simulink model "three_way_newest_1"  (R2025b)
settings: Solver=VariableStepAuto  StartTime=0.0  StopTime=20  RelTol=1e-3
undefined symbols (not defined in the file or in its folder): c, dspblkCoreblockFVToolHelper, gcbh, sfvc784, xck26
libraries: hdlBasic x131, hdlDSPIP x11, simulink x10, hdlUtilities x4, vmcUtilities x1
(part 2 of 2)

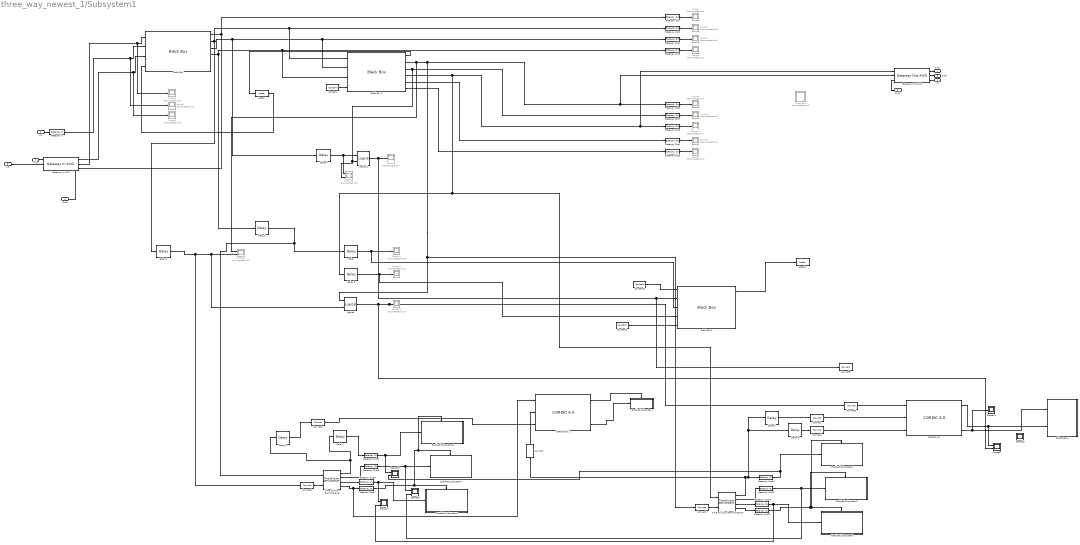
== system three_way_newest_1/Subsystem1 ==
  In1 : Inport
  In2 : Inport  Port=2
  In3 : Inport  Port=3
  In4 : Inport  Port=4
  Assert : hdlBasic/Assert  assert_type=on  type_source=Explicitly  gui_display_data_type=Fixed-point  arith_type=Unsigned  n_bits=1  bin_pt=0  preci_type=Single  exp_width=8  frac_width=24  assert_rate=on  rate_source=Explicitly  period=1/81000  output_port=on  XmcBlockStatus=1  maskContainerNames=group1  block_type=assert  block_config=sysgen:assert_config  block_width=609  block_height=900
  Assert1 : hdlBasic/Assert  assert_type=on  type_source=Explicitly  gui_display_data_type=Fixed-point  arith_type=Unsigned  n_bits=1  bin_pt=0  preci_type=Single  exp_width=8  frac_width=24  assert_rate=on  rate_source=Explicitly  period=1/81000  output_port=on  XmcBlockStatus=1  maskContainerNames=group1  block_type=assert  block_config=sysgen:assert_config  block_width=609  block_height=900
  Black Box : hdlBasic/Black Box  init_code=fir_compiler_0_wrapper_config  sim_method=Vivado Simulator  verbose=off  XmcBlockStatus=1  maskContainerNames=group1  block_type=blackbox2  block_config=sysgen:black_box_config
  Black Box1 : hdlBasic/Black Box  init_code=fir_compiler_1_wrapper_config  sim_method=Vivado Simulator  verbose=off  XmcBlockStatus=1  maskContainerNames=group1  block_type=blackbox2  block_config=sysgen:black_box_config
  Black Box2 : hdlBasic/Black Box  init_code=cordic_0_wrapper_config  sim_method=Vivado Simulator  verbose=off  XmcBlockStatus=1  maskContainerNames=group1  block_type=blackbox2  block_config=sysgen:black_box_config
  "CORDIC 6.0 " : hdlDSPIP/CORDIC 6.0   functional_selection=Translate  architectural_configuration=Parallel  pipelining_mode=Maximum  data_format=SignedFraction  phase_format=Radians  input_width=16  output_width=16  round_mode=Nearest_Even  iterations=0  precision=0  compensation_scaling=BRAM  coarse_rotation=on  aclken=off  aresetn=off  out_tready=off  cartesian_has_tuser=off  cartesian_has_tlast=off  cartesian_tuser_width=1  phase_has_tuser=off  phase_has_tlast=off  phase_tuser_width=1  out_tlast_behv=Null  flow_control=NonBlocking  optimize_goal=Resources  trim_axipin_name=on  simulation_type=hybrid_sim  simulation_model=sysgen:cordic_v6_0  data_path_portlist={'s_axis_cartesian_tdata_imag', 's_axis_cartesian_tdata_real', 's_axis_phase_tdata_phase', 'm_axis_dout_tdata_imag', 'm_axis_dout_tdata_real', 'm_axis_dout_tdata_phase','m_axis_dout_tdata'}  ip_name=CORDIC  ip_version=6.0  dsptool_ready=true  ipcore_usecache=true  ipcore_useipmodelcache=true  wrapper_available=true  port_translation_map={ 'aclken' => 'en', 'aresetn' => 'rst' }  XmcBlockStatus=1  maskContainerNames=group15  block_type=cordic_v6_0  block_config=sysgen:rodinimport_config  block_width=800
  CORDIC 6.0 1 : hdlDSPIP/CORDIC 6.0   functional_selection=Translate  architectural_configuration=Parallel  pipelining_mode=Maximum  data_format=SignedFraction  phase_format=Radians  input_width=16  output_width=16  round_mode=Nearest_Even  iterations=0  precision=0  compensation_scaling=BRAM  coarse_rotation=on  aclken=off  aresetn=off  out_tready=off  cartesian_has_tuser=off  cartesian_has_tlast=off  cartesian_tuser_width=1  phase_has_tuser=off  phase_has_tlast=off  phase_tuser_width=1  out_tlast_behv=Null  flow_control=NonBlocking  optimize_goal=Resources  trim_axipin_name=on  simulation_type=hybrid_sim  simulation_model=sysgen:cordic_v6_0  data_path_portlist={'s_axis_cartesian_tdata_imag', 's_axis_cartesian_tdata_real', 's_axis_phase_tdata_phase', 'm_axis_dout_tdata_imag', 'm_axis_dout_tdata_real', 'm_axis_dout_tdata_phase','m_axis_dout_tdata'}  ip_name=CORDIC  ip_version=6.0  dsptool_ready=true  ipcore_usecache=true  ipcore_useipmodelcache=true  wrapper_available=true  port_translation_map={ 'aclken' => 'en', 'aresetn' => 'rst' }  XmcBlockStatus=1  maskContainerNames=group15  block_type=cordic_v6_0  block_config=sysgen:rodinimport_config  block_width=800
  Constant : hdlBasic/Constant  const=1.0  gui_display_data_type=Boolean  arith_type=Boolean  n_bits=16  bin_pt=14  preci_type=Single  exp_width=8  frac_width=24  explicit_period=off  period=1  XmcBlockStatus=1  maskContainerNames=tabcontainer1  block_type=constant  block_config=sysgen:Constant_config
  Constant1 : hdlBasic/Constant  const=1.0  gui_display_data_type=Boolean  arith_type=Boolean  n_bits=16  bin_pt=14  preci_type=Single  exp_width=8  frac_width=24  explicit_period=off  period=1  XmcBlockStatus=1  maskContainerNames=tabcontainer1  block_type=constant  block_config=sysgen:Constant_config
  Constant2 : hdlBasic/Constant  const=1.0  gui_display_data_type=Boolean  arith_type=Boolean  n_bits=16  bin_pt=14  preci_type=Single  exp_width=8  frac_width=24  explicit_period=off  period=1  XmcBlockStatus=1  maskContainerNames=tabcontainer1  block_type=constant  block_config=sysgen:Constant_config
  Convert{,2,4,7} (4 alike) : hdlBasic/Convert  gui_display_data_type=Fixed-point  arith_type=Signed (2's comp)  n_bits=16  bin_pt=14  float_type=Single  exp_bits=8  fraction_bits=24  quantization="Round  (unbiased: +/- Inf)"  overflow=Saturate  en=off  latency=0  pipeline=off  XmcBlockStatus=1  maskContainerNames=group2  block_type=convert  block_config=sysgen:Convert_config  block_width=595  block_height=885
  Convert{1,3,5..6} (4 alike) : hdlBasic/Convert  gui_display_data_type=Boolean  arith_type=Boolean  n_bits=16  bin_pt=14  float_type=Single  exp_bits=8  fraction_bits=24  quantization=Truncate  overflow=Wrap  en=off  latency=0  pipeline=off  XmcBlockStatus=1  maskContainerNames=group2  block_type=convert  block_config=sysgen:Convert_config  block_width=595  block_height=885
  Delay{,3,5..6} (4 alike) : hdlBasic/Delay  rst=off  en=off  latency=1  reg_retiming=off  XmcBlockStatus=1  maskContainerNames=group1  block_type=delay  block_config=sysgen:Delay_config
  Delay1 : hdlBasic/Delay  rst=off  en=off  latency=30  reg_retiming=off  XmcBlockStatus=1  maskContainerNames=group1  block_type=delay  block_config=sysgen:Delay_config
  Delay2 : hdlBasic/Delay  rst=off  en=off  latency=30  reg_retiming=off  XmcBlockStatus=1  maskContainerNames=group1  block_type=delay  block_config=sysgen:Delay_config
  Delay4 : hdlBasic/Delay  rst=off  en=off  latency=30  reg_retiming=off  XmcBlockStatus=1  maskContainerNames=group1  block_type=delay  block_config=sysgen:Delay_config
  Delay7 : hdlBasic/Delay  rst=off  en=off  latency=267  reg_retiming=off  XmcBlockStatus=1  maskContainerNames=group1  block_type=delay  block_config=sysgen:Delay_config
  Delay8 : hdlBasic/Delay  rst=off  en=off  latency=267  reg_retiming=off  XmcBlockStatus=1  maskContainerNames=group1  block_type=delay  block_config=sysgen:Delay_config
  Enabled Subsystem : Subsystem  TreatAsAtomicUnit=on
  Enabled Subsystem1 : Subsystem  TreatAsAtomicUnit=on
  Enabled Subsystem2 : Subsystem  TreatAsAtomicUnit=on
  Enabled Subsystem3 : Subsystem  TreatAsAtomicUnit=on
  Enabled Subsystem6 : Subsystem  TreatAsAtomicUnit=on
  Enabled Subsystem7 : Subsystem  TreatAsAtomicUnit=on
  Enabled Subsystem8 : Subsystem  TreatAsAtomicUnit=on
  Gateway In : hdlBasic/Gateway In  gui_display_data_type=Boolean  arith_type=Boolean  n_bits=16  bin_pt=14  preci_type=Single  exp_width=8  frac_width=24  rows=1  columns=1  quantization="Round  (unbiased: +/- Inf)"  overflow=Saturate  period=1/81000  UseAsADC=off  ADCChannel='1'  interface=None  automatic_assignment=on  address_offset=hex2dec('00')  intf_name=''  intf_description=''  default_value=0  timing_constraint=None  locs_specified=off  LOCs={}  io_standard={}  inherit_from_input=off  hdl_port=on  XmcBlockStatus=1  maskContainerNames=group4  block_type=gatewayin  block_config=sysgen:gateway_in_config  block_width_w=590  block_height_w=620  block_width=640  block_height=850
  Gateway In AXIS : hdlUtilities/Gateway In AXIS  gui_display_data_type=Fixed-point  arith_type=Signed (2's comp)  n_bits=16  bin_pt=14  preci_type=Custom  exp_width=16  frac_width=24  quantization="Round  (unbiased: +/- Inf)"  overflow=Saturate  bool_to_boolean=off  OutSampleTime=1/81000  block_type=gatewayinaxi  XmcBlockStatus=1
  Gateway Out{,1..13,23..25} (17 alike) : hdlBasic/Gateway Out  inherit_from_input=off  bool_to_boolean=off  hdl_port=on  rows=1  columns=1  UseAsDAC=off  DACChannel='1'  interface=None  automatic_assignment=on  address_offset=hex2dec('00')  intf_name=''  intf_description=''  timing_constraint=None  locs_specified=off  LOCs={}  io_standard={}  XmcBlockStatus=1  maskContainerNames=group4  block_type=gatewayout  block_config=sysgen:gateway_out_config  block_width_w=590  block_height_w=620  block_width=620  block_height=750
  Gateway Out AXIS : hdlUtilities/Gateway Out AXIS  mask_sample_period=1/81000  bool_to_boolean=off  block_type=gatewayoutaxi
  Logical : hdlBasic/Logical  logical_function=AND  inputs=2  en=off  latency=1  precision=Full  arith_type=Unsigned  n_bits=16  bin_pt=0  align_bp=on  overflow=[]  quantization=[]  XmcBlockStatus=1  maskContainerNames=tabcontainer1  block_type=logical  block_config=sysgen:Logical_config
  Logical1 : hdlBasic/Logical  logical_function=AND  inputs=2  en=off  latency=1  precision=Full  arith_type=Unsigned  n_bits=16  bin_pt=0  align_bp=on  overflow=[]  quantization=[]  XmcBlockStatus=1  maskContainerNames=tabcontainer1  block_type=logical  block_config=sysgen:Logical_config
  Scope{,1..12,14,18..19} (16 alike) : Scope  Commented=on
      Scope settings: ActiveDisplayYMinimum=-0.12499999999999997  ActiveDisplayYMaximum=1.125
      Scope1 settings: ActiveDisplayYMinimum=-0.12499999999999997  ActiveDisplayYMaximum=1.125
      Scope10 settings: ActiveDisplayYMinimum=-0.12499999999999997  ActiveDisplayYMaximum=1.125  DataLoggingVariableName=ScopeData12
      Scope11 settings: ActiveDisplayYMinimum=-0.76177978515625  ActiveDisplayYMaximum=0.79644775390625  DataLoggingVariableName=ScopeData13
      Scope12 settings: ActiveDisplayYMinimum=-1.584625244140625  ActiveDisplayYMaximum=1.432037353515625  DataLoggingVariableName=ScopeData8
      Scope14 settings: ActiveDisplayYMinimum=-1.5235595703125  ActiveDisplayYMaximum=1.5928955078125  DataLoggingVariableName=ScopeData20
      Scope18 settings: ActiveDisplayYMinimum=-0.12499999999999997  ActiveDisplayYMaximum=1.125  DataLoggingVariableName=ScopeData21
      Scope19 settings: ActiveDisplayYMinimum=-0.12499999999999997  ActiveDisplayYMaximum=1.125  DataLoggingVariableName=ScopeData22
      Scope2 settings: ActiveDisplayYMinimum=-0.12499999999999997  ActiveDisplayYMaximum=1.125  DataLoggingVariableName=ScopeData2
      Scope3 settings: ActiveDisplayYMinimum=-1.584625244140625  ActiveDisplayYMaximum=1.432037353515625  DataLoggingVariableName=ScopeData3
      Scope4 settings: ActiveDisplayYMinimum=-0.12499999999999997  ActiveDisplayYMaximum=1.125  DataLoggingVariableName=ScopeData4
      Scope5 settings: ActiveDisplayYMinimum=-0.12499999999999997  ActiveDisplayYMaximum=1.125  DataLoggingVariableName=ScopeData5
      Scope6 settings: ActiveDisplayYMinimum=0.9  ActiveDisplayYMaximum=1.1  DataLoggingVariableName=ScopeData9
      Scope7 settings: ActiveDisplayYMinimum=-0.12499999999999997  ActiveDisplayYMaximum=1.125  DataLoggingVariableName=ScopeData10
      Scope8 settings: ActiveDisplayYMinimum=-1.5119476318359375  ActiveDisplayYMaximum=1.7752532958984375  DataLoggingVariableName=ScopeData11
      Scope9 settings: ActiveDisplayYMinimum=-0.12499999999999997  ActiveDisplayYMaximum=1.125  DataLoggingVariableName=ScopeData14
  Scope13 : Scope  Commented=on  NumInputPorts=2
      settings: ActiveDisplayYMinimum=-0.12499999999999997  ActiveDisplayYMaximum=1.125  DataLoggingVariableName=ScopeData7
  Scope{15..17,22} (4 alike) : Scope  NumInputPorts=2
      Scope15 settings: ActiveDisplayYMinimum=-1.06396484375  ActiveDisplayYMaximum=1.06005859375  DataLoggingVariableName=ScopeData16
      Scope16 settings: ActiveDisplayYMinimum=-1.330322265625  ActiveDisplayYMaximum=1.347900390625  DataLoggingVariableName=ScopeData18
      Scope17 settings: ActiveDisplayYMinimum=-1.603485107421875  ActiveDisplayYMaximum=1.601776123046875  DataLoggingVariableName=ScopeData19
      Scope22 settings: ActiveDisplayYMinimum=-0.046630094043887127  ActiveDisplayYMaximum=1.2033699059561129  DataLoggingVariableName=ScopeData25
  Scope20 : Scope  Commented=on  NumInputPorts=2
      settings: ActiveDisplayYMinimum=-0.12499999999999997  ActiveDisplayYMaximum=1.125  DataLoggingVariableName=ScopeData23
  Scope21 : Scope
      settings: ActiveDisplayYMinimum=-0.18955230712890619  ActiveDisplayYMaximum=1.7059707641601562  DataLoggingVariableName=ScopeData24
  Scope23 : Scope
      settings: ActiveDisplayYMinimum=-0.056299574817166853  ActiveDisplayYMaximum=1.1341766156590241  DataLoggingVariableName=ScopeData26
  Subsystem : Subsystem  Commented=on
  Subsystem1 : Subsystem
  Time Division Demultiplexer : hdlBasic/Time Division Demultiplexer  frame_pattern=[1 1 1]  impl_style=Multiple Channel  vin=on  explicit_period=off  period=1  XmcBlockStatus=1  maskContainerNames=group2  block_type=tdd  block_config=sysgen:TDD_config
  Time Division Demultiplexer1 : hdlBasic/Time Division Demultiplexer  frame_pattern=[1 1 1]  impl_style=Multiple Channel  vin=on  explicit_period=off  period=1  XmcBlockStatus=1  maskContainerNames=group2  block_type=tdd  block_config=sysgen:TDD_config
  Out1 : Outport
  Out3 : Outport  Port=2
  Out4 : Outport  Port=3
  Out5 : Outport  Port=4
  wires:
  Gateway In AXIS/3 -> Out5/1
  In3/1 -> Gateway In AXIS/2
  In2/1 -> Gateway Out AXIS/3
  Gateway Out AXIS/1 -> Out1/1
  Gateway Out AXIS/3 -> Out4/1
  In1/1 -> Gateway In AXIS/1
  Gateway Out AXIS/2 -> Out3/1
  In4/1 -> Gateway In/1
  Gateway In AXIS/1 -> Black Box/3, Scope8/1
  Gateway In/1 -> Black Box/2, Scope7/1
  Gateway In AXIS/2 -> Black Box/1, Scope6/1
  Black Box/1 -> Gateway In AXIS/3, Gateway Out/1
  Black Box/2 -> Delay1/1, Black Box1/1, Gateway Out1/1
  Black Box/3 -> Delay4/1, Black Box1/2, Gateway Out2/1
  Black Box/4 -> Delay2/1, Black Box1/3, Gateway Out3/1
  Gateway Out/1 -> Scope/1
  Gateway Out1/1 -> Scope1/1
  Gateway Out2/1 -> Scope2/1
  Gateway Out3/1 -> Scope3/1
  Gateway Out4/1 -> Scope4/1
  Gateway Out5/1 -> Scope5/1
  Black Box1/5 -> Gateway Out4/1
  Black Box1/6 -> Gateway Out5/1
  Gateway Out7/1 -> Scope10/1
  Gateway Out6/1 -> Scope9/1
  Gateway Out8/1 -> Scope11/1
  Black Box1/3 -> Scope20/2, Logical1/2, Gateway Out7/1
  Black Box1/2 -> Scope13/1, Logical/1, Convert1/1, Gateway Out AXIS/2, Gateway Out6/1
  Black Box2/1 -> Assert1/1
  Black Box1/1 -> Assert/1
  Assert/1 -> Black Box/4
  Black Box1/4 -> Delay3/1, Time Division Demultiplexer1/1, Gateway Out AXIS/1, Gateway Out8/1
  Time Division Demultiplexer/1 -> Delay7/1, Delay8/1
  Time Division Demultiplexer/2 -> Gateway Out25/1
  Time Division Demultiplexer/3 -> Gateway Out24/1
  Convert3/1 -> Time Division Demultiplexer/2
  Gateway Out23/1 -> Enabled Subsystem6/1(In1), Scope15/1
  Gateway Out25/1 -> Scope16/1, Enabled Subsystem7/1(In1)
  Gateway Out24/1 -> Scope17/1, Enabled Subsystem8/1(In1)
  Time Division Demultiplexer/4 -> CORDIC 6.0 1/1, Gateway Out9/1
  Time Division Demultiplexer1/2 -> Gateway Out12/1
  Time Division Demultiplexer1/1 -> Delay5/1, Delay6/1, Gateway Out10/1, Convert7/1
  Convert1/1 -> Time Division Demultiplexer1/2
  Time Division Demultiplexer1/4 -> Gateway Out13/1
  Time Division Demultiplexer1/3 -> Gateway Out11/1
  Gateway Out11/1 -> Scope17/2, Enabled Subsystem3/1(In1)
  Gateway Out12/1 -> Scope16/2, Enabled Subsystem2/1(In1)
  Gateway Out10/1 -> Enabled Subsystem1/1(In1), Scope15/2
  Gateway Out13/1 -> Enabled Subsystem1/Enable, Enabled Subsystem3/Enable, Enabled Subsystem2/Enable
  Delay3/1 -> Black Box2/4, Scope14/1
  Delay/1 -> Black Box2/3, Scope12/1
  Delay4/1 -> Scope20/1, Logical1/1
  Logical1/1 -> Convert5/1, Black Box2/2, Scope19/1
  Constant1/1 -> Black Box2/5
  Constant/1 -> Black Box1/4
  Logical/1 -> Convert6/1, Scope18/1, Scope22/2
  Delay5/1 -> Convert/1
  Delay6/1 -> Convert4/1
  Delay2/1 -> Delay/1, Time Division Demultiplexer/1
  Delay1/1 -> Convert3/1, Logical/2, Scope13/2
  Convert4/1 -> "CORDIC 6.0 "/3
  Convert/1 -> "CORDIC 6.0 "/2
  Convert6/1 -> "CORDIC 6.0 "/1
  Constant2/1 -> Black Box2/1
  "CORDIC 6.0 "/3 -> Scope21/1, Subsystem1/1(In1)
  "CORDIC 6.0 "/1 -> Scope22/1, Subsystem1/2(In2)
  Gateway Out9/1 -> Enabled Subsystem6/Enable, Enabled Subsystem7/Enable, Enabled Subsystem8/Enable
  CORDIC 6.0 1/3 -> Enabled Subsystem/1(In1)
  Convert2/1 -> CORDIC 6.0 1/3
  CORDIC 6.0 1/1 -> Enabled Subsystem/Enable
  Delay7/1 -> Gateway Out23/1
  Delay8/1 -> Convert2/1
  Convert7/1 -> CORDIC 6.0 1/2

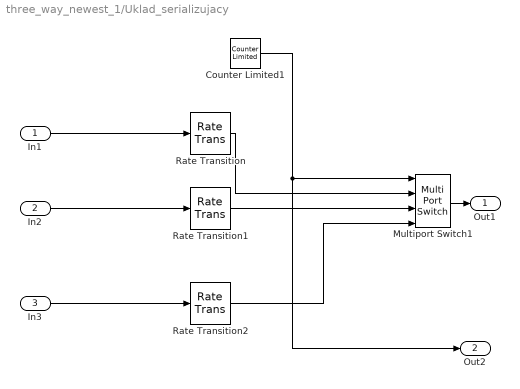
== system three_way_newest_1/Uklad_serializujacy ==
  In1 : Inport
  In2 : Inport  Port=2
  In3 : Inport  Port=3
  Counter Limited1 : simulink/Sources/Counter Limited  uplimit=2  tsamp=1/81000
  Multiport Switch1 : MultiPortSwitch  DataPortOrder=Zero-based contiguous  zeroidx=on  SaturateOnIntegerOverflow=off  InputSameDT=off
  Rate Transition : RateTransition  OutPortSampleTime=1/81000
  Rate Transition1 : RateTransition  OutPortSampleTime=1/81000
  Rate Transition2 : RateTransition  OutPortSampleTime=1/81000
  Out1 : Outport
  Out2 : Outport  Port=2
  wires:
  In1/1 -> Rate Transition/1
  Rate Transition2/1 -> Multiport Switch1/4
  Counter Limited1/1 -> Out2/1, Multiport Switch1/1
  Rate Transition1/1 -> Multiport Switch1/3
  In2/1 -> Rate Transition1/1
  Rate Transition/1 -> Multiport Switch1/2
  In3/1 -> Rate Transition2/1
  Multiport Switch1/1 -> Out1/1

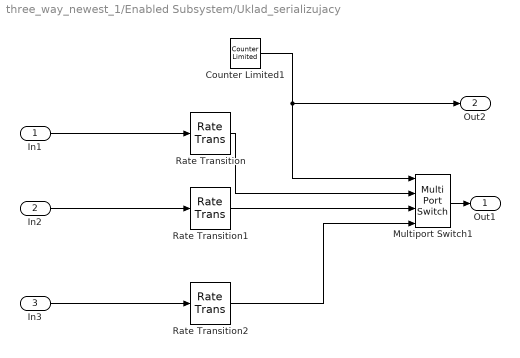
== system three_way_newest_1/Enabled Subsystem/Uklad_serializujacy ==
  In1 : Inport
  In2 : Inport  Port=2
  In3 : Inport  Port=3
  Counter Limited1 : simulink/Sources/Counter Limited  uplimit=2  tsamp=1/81000
  Multiport Switch1 : MultiPortSwitch  DataPortOrder=Zero-based contiguous  zeroidx=on  SaturateOnIntegerOverflow=off  InputSameDT=off
  Rate Transition : RateTransition  OutPortSampleTime=1/81000
  Rate Transition1 : RateTransition  OutPortSampleTime=1/81000
  Rate Transition2 : RateTransition  OutPortSampleTime=1/81000
  Out1 : Outport
  Out2 : Outport  Port=2
  wires:
  In1/1 -> Rate Transition/1
  Rate Transition2/1 -> Multiport Switch1/4
  Counter Limited1/1 -> Out2/1, Multiport Switch1/1
  Rate Transition1/1 -> Multiport Switch1/3
  In2/1 -> Rate Transition1/1
  Rate Transition/1 -> Multiport Switch1/2
  In3/1 -> Rate Transition2/1
  Multiport Switch1/1 -> Out1/1

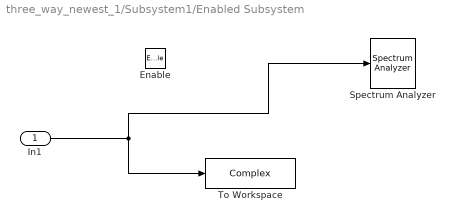
== system three_way_newest_1/Subsystem1/Enabled Subsystem ==
  In1 : Inport
  Enable : EnablePort
  Spectrum Analyzer : SpectrumAnalyzer  WindowPosition=[880.000000,470.000000,800.000000,500.000000,]  ScopeFrameLocation=window  SampleRateSource=Property  SampleRate=27000  WindowInvariantSamplesPerUpdate=on  Span=27000  StartFrequency=-13500  StopFrequency=13500  YLimits=[-67.5454 13.052]
  To Workspace : ToWorkspace  VariableName=Complex  SampleTime=-1
  wires:
  In1/1 -> To Workspace/1, Spectrum Analyzer/1

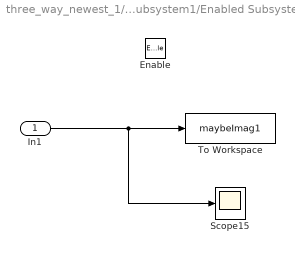
== system three_way_newest_1/Subsystem1/Enabled Subsystem1 ==
  In1 : Inport
  Enable : EnablePort
  Scope15 : Scope
      settings: ActiveDisplayYMinimum=-1  ActiveDisplayYMaximum=1  DataLoggingVariableName=ScopeData17
  To Workspace : ToWorkspace  VariableName=maybeImag1  SampleTime=-1
  wires:
  In1/1 -> Scope15/1, To Workspace/1

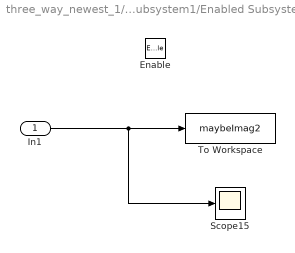
== system three_way_newest_1/Subsystem1/Enabled Subsystem2 ==
  In1 : Inport
  Enable : EnablePort
  Scope15 : Scope
      settings: ActiveDisplayYMinimum=-1  ActiveDisplayYMaximum=1  DataLoggingVariableName=ScopeData17
  To Workspace : ToWorkspace  VariableName=maybeImag2  SampleTime=-1
  wires:
  In1/1 -> Scope15/1, To Workspace/1

== system three_way_newest_1/Subsystem1/Enabled Subsystem3 ==
  In1 : Inport
  Enable : EnablePort
  Scope15 : Scope
      settings: ActiveDisplayYMinimum=-1  ActiveDisplayYMaximum=1  DataLoggingVariableName=ScopeData17
  To Workspace : ToWorkspace  VariableName=maybeImag3  SampleTime=-1
  wires:
  In1/1 -> Scope15/1, To Workspace/1

== system three_way_newest_1/Subsystem1/Enabled Subsystem6 ==
  In1 : Inport
  Enable : EnablePort
  Scope15 : Scope
      settings: ActiveDisplayYMinimum=-1  ActiveDisplayYMaximum=1  DataLoggingVariableName=ScopeData17
  To Workspace : ToWorkspace  VariableName=maybeReal1  SampleTime=-1
  wires:
  In1/1 -> Scope15/1, To Workspace/1

== system three_way_newest_1/Subsystem1/Enabled Subsystem7 ==
  In1 : Inport
  Enable : EnablePort
  Scope15 : Scope
      settings: ActiveDisplayYMinimum=-1  ActiveDisplayYMaximum=1  DataLoggingVariableName=ScopeData17
  To Workspace : ToWorkspace  VariableName=maybeReal2  SampleTime=-1
  wires:
  In1/1 -> Scope15/1, To Workspace/1

== system three_way_newest_1/Subsystem1/Enabled Subsystem8 ==
  In1 : Inport
  Enable : EnablePort
  Scope15 : Scope
      settings: ActiveDisplayYMinimum=-1  ActiveDisplayYMaximum=1  DataLoggingVariableName=ScopeData17
  To Workspace : ToWorkspace  VariableName=maybeReal3  SampleTime=-1
  wires:
  In1/1 -> Scope15/1, To Workspace/1

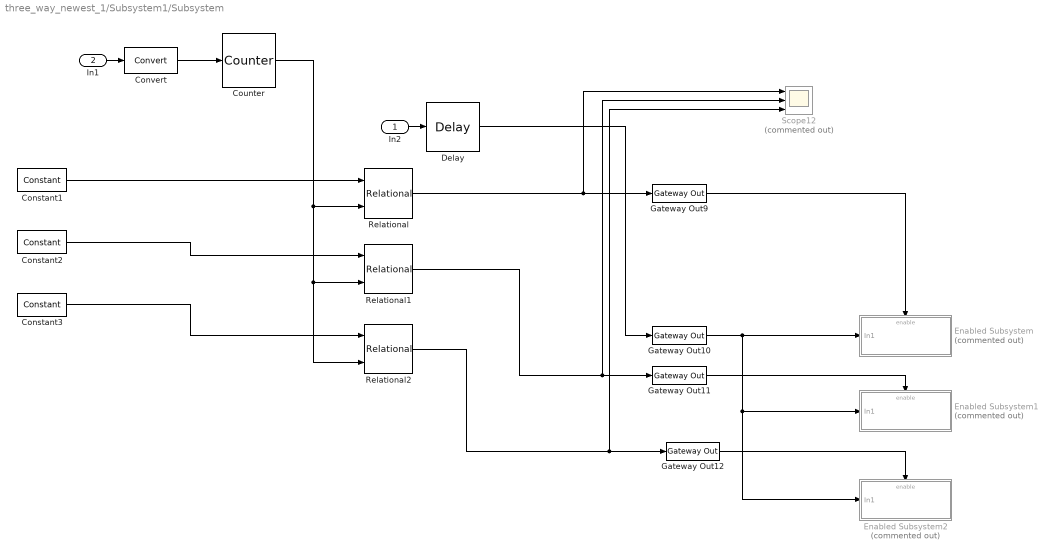
== system three_way_newest_1/Subsystem1/Subsystem ==
  In2 : Inport
  In1 : Inport  Port=2
  Constant1 : hdlBasic/Constant  const=0  gui_display_data_type=Fixed-point  arith_type=Unsigned  n_bits=2  bin_pt=0  preci_type=Single  exp_width=8  frac_width=24  explicit_period=off  period=1  XmcBlockStatus=1  maskContainerNames=tabcontainer1  block_type=constant  block_config=sysgen:Constant_config
  Constant2 : hdlBasic/Constant  const=1  gui_display_data_type=Fixed-point  arith_type=Unsigned  n_bits=2  bin_pt=0  preci_type=Single  exp_width=8  frac_width=24  explicit_period=off  period=1  XmcBlockStatus=1  maskContainerNames=tabcontainer1  block_type=constant  block_config=sysgen:Constant_config
  Constant3 : hdlBasic/Constant  const=2  gui_display_data_type=Fixed-point  arith_type=Unsigned  n_bits=2  bin_pt=0  preci_type=Single  exp_width=8  frac_width=24  explicit_period=off  period=1  XmcBlockStatus=1  maskContainerNames=tabcontainer1  block_type=constant  block_config=sysgen:Constant_config
  Convert : hdlBasic/Convert  gui_display_data_type=Boolean  arith_type=Boolean  n_bits=16  bin_pt=14  float_type=Single  exp_bits=8  fraction_bits=24  quantization=Truncate  overflow=Wrap  en=off  latency=1  pipeline=off  XmcBlockStatus=1  maskContainerNames=group2  block_type=convert  block_config=sysgen:Convert_config  block_width=595  block_height=885
  Counter : hdlBasic/Counter  cnt_type=Count limited  cnt_to=2  operation=Up  start_count=0  cnt_by_val=1  arith_type=Unsigned  n_bits=2  bin_pt=0  load_pin=off  rst=off  en=on  explicit_period=Explicit  period=1/81000  use_behavioral_HDL=off  implementation=Fabric  XmcBlockStatus=1  maskContainerNames=group1  block_type=counter  block_config=sysgen:Counter_config  block_width=531  block_height=1023
  Delay : hdlBasic/Delay  rst=off  en=off  latency=3  reg_retiming=off  XmcBlockStatus=1  maskContainerNames=group1  block_type=delay  block_config=sysgen:Delay_config
  Enabled Subsystem : Subsystem  Commented=on  TreatAsAtomicUnit=on
  Enabled Subsystem1 : Subsystem  Commented=on  TreatAsAtomicUnit=on
  Enabled Subsystem2 : Subsystem  Commented=on  TreatAsAtomicUnit=on
  Gateway Out{9..12} (4 alike) : hdlBasic/Gateway Out  inherit_from_input=off  bool_to_boolean=off  hdl_port=on  rows=1  columns=1  UseAsDAC=off  DACChannel='1'  interface=None  automatic_assignment=on  address_offset=hex2dec('00')  intf_name=''  intf_description=''  timing_constraint=None  locs_specified=off  LOCs={}  io_standard={}  XmcBlockStatus=1  maskContainerNames=group4  block_type=gatewayout  block_config=sysgen:gateway_out_config  block_width_w=590  block_height_w=620  block_width=620  block_height=750
  Relational : hdlBasic/Relational  mode=a=b  op_type=Bool  en=off  latency=1  XmcBlockStatus=1  maskContainerNames=tabcontainer1  block_type=relational  block_config=sysgen:Relational_config
  Relational1 : hdlBasic/Relational  mode=a=b  op_type=Bool  en=off  latency=1  XmcBlockStatus=1  maskContainerNames=tabcontainer1  block_type=relational  block_config=sysgen:Relational_config
  Relational2 : hdlBasic/Relational  mode=a=b  op_type=Bool  en=off  latency=1  XmcBlockStatus=1  maskContainerNames=tabcontainer1  block_type=relational  block_config=sysgen:Relational_config
  Scope12 : Scope  Commented=on  NumInputPorts=3
      settings: ActiveDisplayYMinimum=-0.49052241358768922  ActiveDisplayYMaximum=1.3562968911486397  DataLoggingVariableName=ScopeData6
  wires:
  Gateway Out12/1 -> Enabled Subsystem2/Enable
  Relational2/1 -> Scope12/3, Gateway Out12/1
  Gateway Out9/1 -> Enabled Subsystem/Enable
  Constant2/1 -> Relational1/1
  Gateway Out10/1 -> Enabled Subsystem2/1(In1), Enabled Subsystem1/1(In1), Enabled Subsystem/1(In1)
  In1/1 -> Convert/1
  Counter/1 -> Relational/2, Relational1/2, Relational2/2
  Relational1/1 -> Scope12/2, Gateway Out11/1
  Relational/1 -> Scope12/1, Gateway Out9/1
  Constant1/1 -> Relational/1
  Gateway Out11/1 -> Enabled Subsystem1/Enable
  Constant3/1 -> Relational2/1
  Delay/1 -> Gateway Out10/1
  Convert/1 -> Counter/1
  In2/1 -> Delay/1

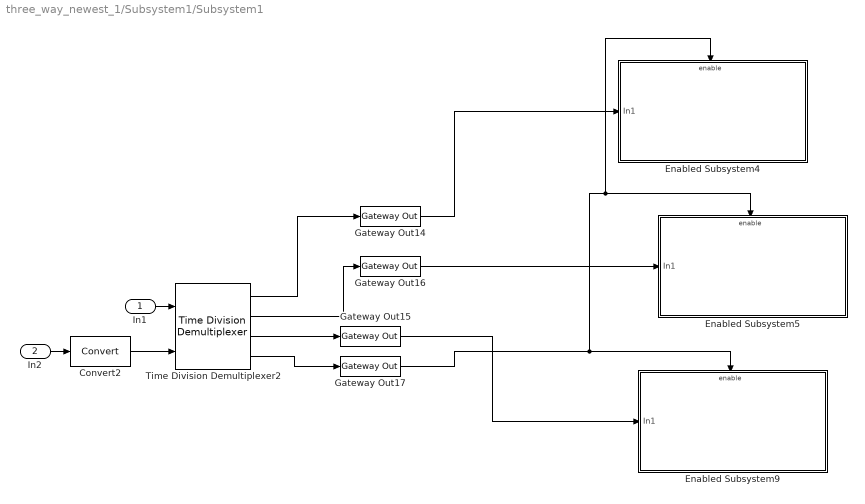
== system three_way_newest_1/Subsystem1/Subsystem1 ==
  In1 : Inport
  In2 : Inport  Port=2
  Convert2 : hdlBasic/Convert  gui_display_data_type=Boolean  arith_type=Boolean  n_bits=16  bin_pt=14  float_type=Single  exp_bits=8  fraction_bits=24  quantization=Truncate  overflow=Wrap  en=off  latency=0  pipeline=off  XmcBlockStatus=1  maskContainerNames=group2  block_type=convert  block_config=sysgen:Convert_config  block_width=595  block_height=885
  Enabled Subsystem4 : Subsystem  TreatAsAtomicUnit=on
  Enabled Subsystem5 : Subsystem  TreatAsAtomicUnit=on
  Enabled Subsystem9 : Subsystem  TreatAsAtomicUnit=on
  Gateway Out{14..17} (4 alike) : hdlBasic/Gateway Out  inherit_from_input=off  bool_to_boolean=off  hdl_port=on  rows=1  columns=1  UseAsDAC=off  DACChannel='1'  interface=None  automatic_assignment=on  address_offset=hex2dec('00')  intf_name=''  intf_description=''  timing_constraint=None  locs_specified=off  LOCs={}  io_standard={}  XmcBlockStatus=1  maskContainerNames=group4  block_type=gatewayout  block_config=sysgen:gateway_out_config  block_width_w=590  block_height_w=620  block_width=620  block_height=750
  Time Division Demultiplexer2 : hdlBasic/Time Division Demultiplexer  frame_pattern=[1 1 1]  impl_style=Multiple Channel  vin=on  explicit_period=off  period=1  XmcBlockStatus=1  maskContainerNames=group2  block_type=tdd  block_config=sysgen:TDD_config
  wires:
  Time Division Demultiplexer2/1 -> Gateway Out14/1
  Gateway Out15/1 -> Enabled Subsystem9/1(In1)
  Gateway Out17/1 -> Enabled Subsystem4/Enable, Enabled Subsystem5/Enable, Enabled Subsystem9/Enable
  Gateway Out16/1 -> Enabled Subsystem5/1(In1)
  Gateway Out14/1 -> Enabled Subsystem4/1(In1)
  Time Division Demultiplexer2/4 -> Gateway Out17/1
  Time Division Demultiplexer2/3 -> Gateway Out15/1
  Convert2/1 -> Time Division Demultiplexer2/2
  Time Division Demultiplexer2/2 -> Gateway Out16/1
  In1/1 -> Time Division Demultiplexer2/1
  In2/1 -> Convert2/1

== system three_way_newest_1/Subsystem1/Subsystem/Enabled Subsystem ==
  In1 : Inport
  Enable : EnablePort
  To Workspace : ToWorkspace  VariableName=x  SampleTime=-1
  wires:
  In1/1 -> To Workspace/1

== system three_way_newest_1/Subsystem1/Subsystem/Enabled Subsystem1 ==
  In1 : Inport
  Enable : EnablePort
  To Workspace : ToWorkspace  VariableName=y  SampleTime=-1
  wires:
  In1/1 -> To Workspace/1

== system three_way_newest_1/Subsystem1/Subsystem/Enabled Subsystem2 ==
  In1 : Inport
  Enable : EnablePort
  To Workspace : ToWorkspace  VariableName=z  SampleTime=-1
  wires:
  In1/1 -> To Workspace/1

== system three_way_newest_1/Subsystem1/Subsystem1/Enabled Subsystem4 ==
  In1 : Inport
  Enable : EnablePort
  Scope15 : Scope
      settings: ActiveDisplayYMinimum=-1  ActiveDisplayYMaximum=1  DataLoggingVariableName=ScopeData17
  To Workspace : ToWorkspace  VariableName=maybeComplex1  SampleTime=-1
  wires:
  In1/1 -> Scope15/1, To Workspace/1

== system three_way_newest_1/Subsystem1/Subsystem1/Enabled Subsystem5 ==
  In1 : Inport
  Enable : EnablePort
  Scope15 : Scope
      settings: ActiveDisplayYMinimum=-1  ActiveDisplayYMaximum=1  DataLoggingVariableName=ScopeData17
  To Workspace : ToWorkspace  VariableName=maybeComplex2  SampleTime=-1
  wires:
  In1/1 -> Scope15/1, To Workspace/1

== system three_way_newest_1/Subsystem1/Subsystem1/Enabled Subsystem9 ==
  In1 : Inport
  Enable : EnablePort
  Scope15 : Scope
      settings: ActiveDisplayYMinimum=-1  ActiveDisplayYMaximum=1  DataLoggingVariableName=ScopeData17
  To Workspace : ToWorkspace  VariableName=maybeComplex3  SampleTime=-1
  wires:
  In1/1 -> Scope15/1, To Workspace/1
